simulink model "estimator_poremecaja"  (R2025a)
settings: Solver=VariableStepAuto  StartTime=0.0  StopTime=10.0  RelTol=1e-3
values from neighbouring files (symbols this model uses):
  A = [0, -1; 1, 1]    [d4.m]
  Aw = 0    [d4.m]
  B = [1; 0]    [d4.m]
  C = [0, 1]    [d4.m]
  Cw = 1    [d4.m]
  K = acker(A, B, p_sistem)    [d4.m]
  kr = 1 / dcgain(s * G0 / s)    [d4.m]
  Lw = L(3)    [d4.m]
  Lx = L(1:2)    [d4.m]
  R = 5    [d4.m]
settings Model: Creator=Korisnik  LastModifiedBy=Korisnik

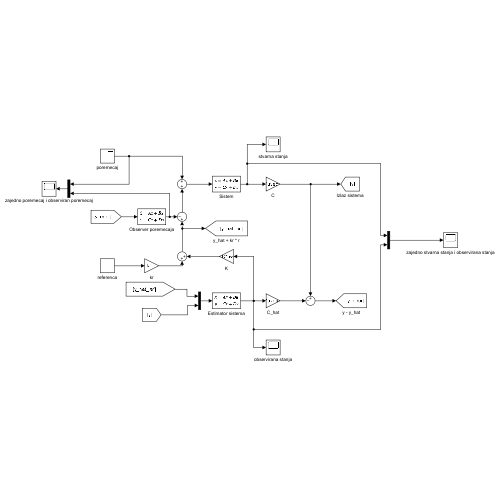
[thumbnail: Simulink's stored preview of the top-level diagram]
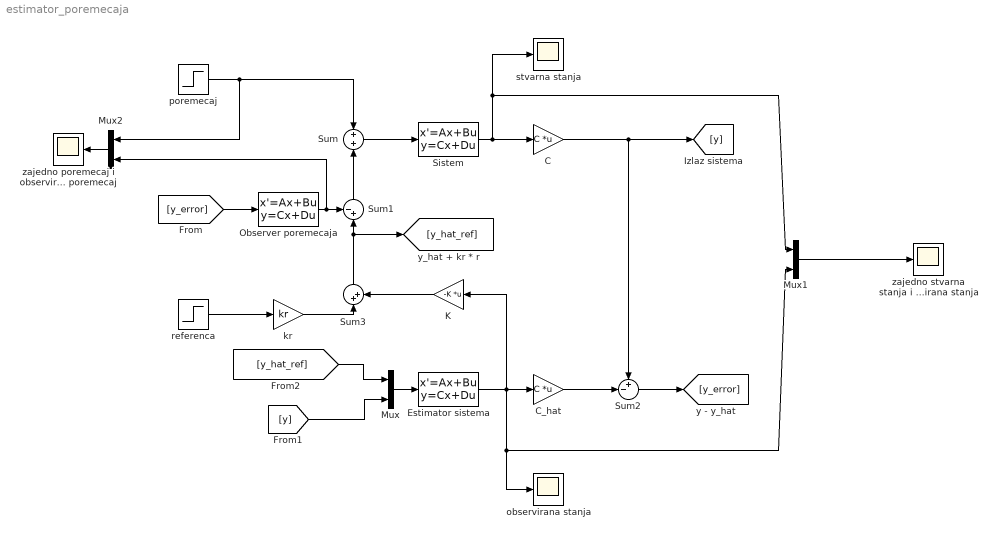
== system estimator_poremecaja ==
  C : Gain  Gain=C  Multiplication=Matrix(K*u) (u vector)
  C_hat : Gain  Gain=C  Multiplication=Matrix(K*u) (u vector)
  Estimator sistema : StateSpace  A=A - Lx * C  B=[B, Lx]  C=[1, 0; 0, 1]  D=[0, 0; 0, 0]  InitialCondition=0
  K : Gain  Gain=-K  Multiplication=Matrix(K*u) (u vector)
  Mux : Mux  Inputs=2
  Mux1 : Mux  Inputs=2
  Mux2 : Mux  Inputs=2
  Observer poremecaja : StateSpace  A=Aw  B=Lw  C=Cw  D=0  InitialCondition=0
  Sistem : StateSpace  A=A  B=B  C=[1, 0; 0, 1]  D=[0; 0]  InitialCondition=[-2; -2]
  Sum : Sum  Inputs=+|+
  Sum1 : Sum  Inputs=-+|
  Sum2 : Sum  Inputs=+-|
  Sum3 : Sum  Inputs=|++
  kr : Gain  Gain=kr
  observirana stanja : Scope
      settings: ActiveDisplayYMinimum=-1  ActiveDisplayYMaximum=1
  poremecaj : Step  Time=0  After=3  SampleTime=0
  referenca : Step  Time=0  After=R  SampleTime=0
  stvarna stanja : Scope
      settings: ActiveDisplayYMinimum=-1  ActiveDisplayYMaximum=1
  zajedno poremecaj i observiran poremecaj : Scope
      settings: ActiveDisplayYMinimum=-21.727813453708386  ActiveDisplayYMaximum=8.5343863270281819  DataLoggingVariableName=ScopeData3
  zajedno stvarna stanja i observirana stanja : Scope
      settings: ActiveDisplayYMinimum=-28.202573148309803  ActiveDisplayYMaximum=27.626513688274084  DataLoggingVariableName=ScopeData2
  wires:
  [y_hat_ref] -> Mux/1
  Sum2/1 -> [y_error]
  Sistem/1 -> C/1, Mux1/1, stvarna stanja/1
  poremecaj/1 -> Mux2/1, Sum/1
  Sum/1 -> Sistem/1
  Estimator sistema/1 -> Mux1/2, observirana stanja/1, K/1, C_hat/1
  [y_error] -> Observer poremecaja/1
  Sum3/1 -> [y_hat_ref], Sum1/2
  kr/1 -> Sum3/1
  Sum1/1 -> Sum/2
  [y] -> Mux/2
  K/1 -> Sum3/2
  Mux/1 -> Estimator sistema/1
  C_hat/1 -> Sum2/2
  C/1 -> Sum2/1, [y]
  Observer poremecaja/1 -> Mux2/2, Sum1/1
  referenca/1 -> kr/1
  Mux1/1 -> zajedno stvarna stanja i observirana stanja/1
  Mux2/1 -> zajedno poremecaj i observiran poremecaj/1
